simulink model "LinearCompetitiveModel"  (R2023b)
settings: Solver=FixedStepAuto  StartTime=0.0  StopTime=inf  RelTol=1e-3
undefined symbols (not defined in the file or in its folder): DiscIntNeverNeededParam
libraries: arduinolib x14, simulink x12, mobileRoboticsTrainingLib x1, arduinosensorlib x1
settings Model: ExtModeTrigDuration=2  Creator=cameronclark  LastModifiedBy=cameronclark
settings OptimizationCC: EnhancedBackFolding=on  PassReuseOutputArgsAs=Individual arguments  ZeroExternalMemoryAtStartup=off  ZeroInternalMemoryAtStartup=off  MaxStackSize=64  OptimizeBlockOrder=speed  DifferentSizesBufferReuse=on  OptimizationCustomize=off  EfficientTunableParamExpr=on
settings DebuggingCC: ParameterTunabilityLossMsg=error
settings HardwareCC: ProdBitPerPointer=32  ProdBitPerSizeT=32  ProdBitPerPtrDiffT=32  ProdLargestAtomicInteger=Long  ProdLargestAtomicFloat=Double  ProdWordSize=32  ProdHWDeviceType=ARM Compatible->ARM Cortex  UseEmbeddedCoderFeatures=off  UseSimulinkCoderFeatures=off
settings SFSimCC: MATLABDynamicMemAlloc=off
settings RTWCC: Description=Embedded Coder  SystemTargetFile=ert.tlc  HardwareBoard=Arduino Nano 33 IoT  TemplateMakefile=ert_default_tmf  Toolchain=Arduino ARM  BuildConfiguration=Faster Runs
settings CodeAppCC: ForceParamTrailComments=on  IgnoreCustomStorageClasses=off  OperatorAnnotations=on  SimulinkDataObjDesc=on  SFDataObjDesc=on  InsertBlockDesc=on
settings ERTTargetCC: SupportContinuousTime=on  SupportNonInlinedSFcns=on  SupportVariableSizeSignals=on  ExtModeTransport=3  ExtModeStaticAlloc=on  ExtModeAutomaticAllocSize=off  ExtModeStaticAllocSize=8192  ExtModeMexFile=ext_xcp  ExtModeIntrfLevel=Level2 - Open

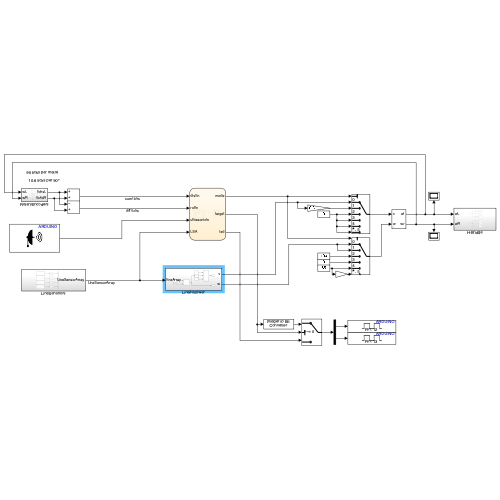
[thumbnail: Simulink's stored preview of the top-level diagram]
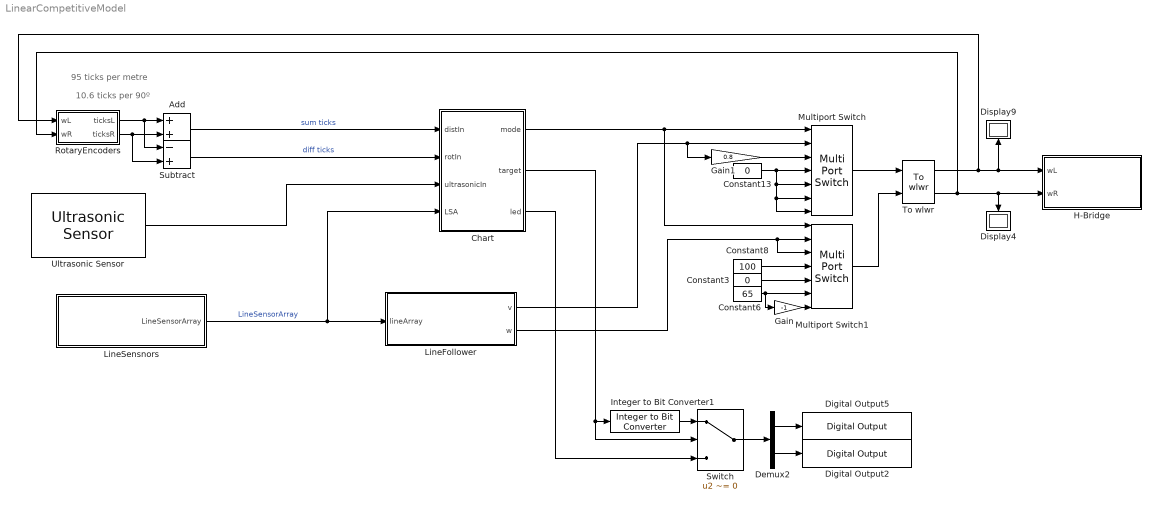
== system LinearCompetitiveModel ==
  note: 95 ticks per metre
  note: 10.6 ticks per 90º
  Add : Sum
  Chart : Stateflow chart  TreatAsAtomicUnit=on
  Constant13 : Constant  Value=0
  Constant3 : Constant  Value=0
  Constant6 : Constant  Value=65
  Constant8 : Constant  Value=100
  Demux2 : Demux  Outputs=2
  Digital Output2 : arduinolib/Digital Output  pinNumber=13  Direction=output  blockPlatform=arduino
  Digital Output5 : arduinolib/Digital Output  pinNumber=12  Direction=output  blockPlatform=arduino
  Display4 : Display
  Display9 : Display
  Gain : Gain  Gain=-1
  Gain1 : Gain  Gain=0.8
  H-Bridge : Subsystem
  Integer to Bit Converter1 : simulink/Logic and Bit Operations/Integer to Bit Converter  nbits=2  signedInputValues=Unsigned  bitOrder=MSB first  outDtype=Inherit via internal rule
  LineFollower : Subsystem
  LineSensnors : Subsystem
  Multiport Switch : MultiPortSwitch  DataPortOrder=Zero-based contiguous  Inputs=6  DataPortIndices={0,1,3,4}  zeroidx=on  SaturateOnIntegerOverflow=off
  Multiport Switch1 : MultiPortSwitch  DataPortOrder=Zero-based contiguous  Inputs=6  DataPortIndices={0,1,3,4}  zeroidx=on  SaturateOnIntegerOverflow=off  InputSameDT=off
  RotaryEncoders : Subsystem
  Subtract : Sum  Inputs=-+
  Switch : Switch  Criteria=u2 ~= 0  SaturateOnIntegerOverflow=off  InputSameDT=off
  To wlwr : mobileRoboticsTrainingLib/To wlwr  axleLength=0.1  wheelR=0.05
      link override change parameters: Gain=[1 -axleLength/2;1 axleLength/2]
  Ultrasonic Sensor : arduinosensorlib/Ultrasonic Sensor  NumSignalPins=2  TrigPin=8  EchoPin=11  SignalPin=3  SampleTime_=0.1  blockPlatform=ARDUINO
  wires:
  RotaryEncoders/2(ticksR) -> Subtract/2, Add/2
  Subtract/1 -> Chart/2(rotIn)  "diff ticks"
  Multiport Switch/1 -> To wlwr/1
  To wlwr/2 -> RotaryEncoders/2(wR), H-Bridge/2(wR), Display4/1
  LineSensnors/1(LineSensorArray) -> LineFollower/1(lineArray), Chart/4(LSA)  "LineSensorArray"
  Constant8/1 -> Multiport Switch1/4
  Multiport Switch1/1 -> To wlwr/2
  Constant6/1 -> Gain/1, Multiport Switch1/6
  LineFollower/1(v) -> Multiport Switch/2, Gain1/1
  Gain/1 -> Multiport Switch1/7
  RotaryEncoders/1(ticksL) -> Subtract/1, Add/1
  Chart/1(mode) -> Multiport Switch/1, Multiport Switch1/1
  Constant3/1 -> Multiport Switch1/5
  LineFollower/2(w) -> Multiport Switch1/2, Multiport Switch1/3
  Ultrasonic Sensor/1 -> Chart/3(ultrasonicIn)
  Constant13/1 -> Multiport Switch/7, Multiport Switch/6, Multiport Switch/5, Multiport Switch/4
  To wlwr/1 -> RotaryEncoders/1(wL), H-Bridge/1(wL), Display9/1
  Add/1 -> Chart/1(distIn)  "sum ticks"
  Demux2/2 -> Digital Output2/1
  Demux2/1 -> Digital Output5/1
  Switch/1 -> Demux2/1
  Gain1/1 -> Multiport Switch/3
  Chart/2(target) -> Integer to Bit Converter1/1, Switch/2
  Chart/3(led) -> Switch/3
  Integer to Bit Converter1/1 -> Switch/1

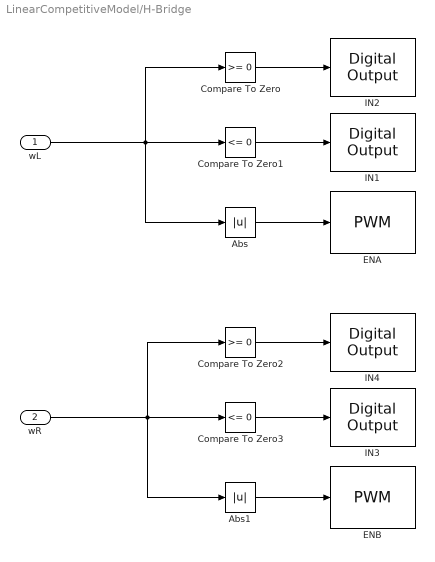
== system LinearCompetitiveModel/H-Bridge ==
  wL : Inport
  wR : Inport  Port=2
  Abs : Abs  SaturateOnIntegerOverflow=off
  Abs1 : Abs  SaturateOnIntegerOverflow=off
  Compare To Zero : simulink/Logic and Bit Operations/Compare To Zero  relop=>=  OutDataTypeStr=boolean
  Compare To Zero1 : simulink/Logic and Bit Operations/Compare To Zero  relop=<=  OutDataTypeStr=boolean
  Compare To Zero2 : simulink/Logic and Bit Operations/Compare To Zero  relop=>=  OutDataTypeStr=boolean
  Compare To Zero3 : simulink/Logic and Bit Operations/Compare To Zero  relop=<=  OutDataTypeStr=boolean
  ENA : arduinolib/PWM  pinNumber=4  frequencyType=Default  desiredFrequency=490.2  achievableFrequency=490.2
  ENB : arduinolib/PWM  pinNumber=5  frequencyType=Default  desiredFrequency=490.2  achievableFrequency=490.2
  IN1 : arduinolib/Digital Output  pinNumber=2  Direction=output  blockPlatform=arduino
  IN2 : arduinolib/Digital Output  pinNumber=3  Direction=output  blockPlatform=arduino
  IN3 : arduinolib/Digital Output  pinNumber=6  Direction=output  blockPlatform=arduino
  IN4 : arduinolib/Digital Output  pinNumber=7  Direction=output  blockPlatform=arduino
  wires:
  Compare To Zero1/1 -> IN1/1
  Compare To Zero/1 -> IN2/1
  Abs1/1 -> ENB/1
  Compare To Zero3/1 -> IN3/1
  Compare To Zero2/1 -> IN4/1
  wL/1 -> Compare To Zero/1, Compare To Zero1/1, Abs/1
  Abs/1 -> ENA/1
  wR/1 -> Compare To Zero2/1, Compare To Zero3/1, Abs1/1

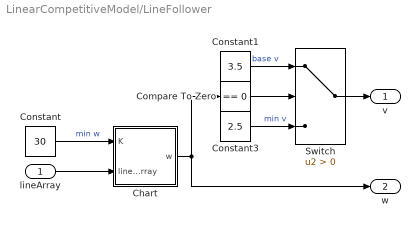
== system LinearCompetitiveModel/LineFollower ==
  lineArray : Inport
  Chart : Stateflow chart  TreatAsAtomicUnit=on
  Compare To Zero : simulink/Logic and Bit Operations/Compare To Zero  relop===  OutDataTypeStr=boolean
  Constant : Constant  Value=30
  Constant1 : Constant  Value=3.5
  Constant3 : Constant  Value=2.5
  Switch : Switch  Criteria=u2 > Threshold  SaturateOnIntegerOverflow=off  InputSameDT=off
  v : Outport
  w : Outport  Port=2
  wires:
  Constant1/1 -> Switch/1  "base v"
  Chart/1(w) -> Compare To Zero/1, w/1
  Constant3/1 -> Switch/3  "min v"
  Switch/1 -> v/1
  lineArray/1 -> Chart/2(lineArray)
  Compare To Zero/1 -> Switch/2
  Constant/1 -> Chart/1(K)  "min w"

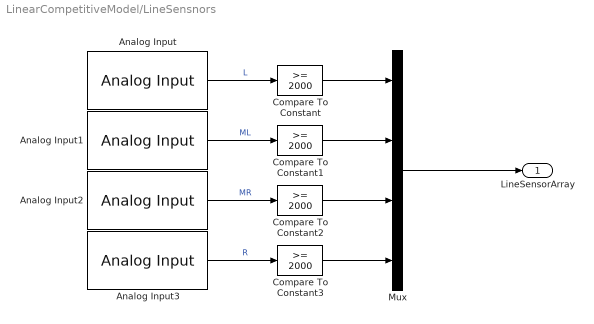
== system LinearCompetitiveModel/LineSensnors ==
  Analog Input : arduinolib/Analog Input  pinNumber=7  ReadResultsOnly=off  ConversionTriggerSource=Software  ExternalTriggerType=uint32( 0 )  OutputDataType=uint16  EnableConversionCompleteNotify=off  EnableOuputStatus=off  SampleTime=-1  blockPlatform=arduino
  Analog Input1 : arduinolib/Analog Input  pinNumber=6  ReadResultsOnly=off  ConversionTriggerSource=Software  ExternalTriggerType=uint32( 0 )  OutputDataType=uint16  EnableConversionCompleteNotify=off  EnableOuputStatus=off  SampleTime=-1  blockPlatform=arduino
  Analog Input2 : arduinolib/Analog Input  pinNumber=3  ReadResultsOnly=off  ConversionTriggerSource=Software  ExternalTriggerType=uint32( 0 )  OutputDataType=uint16  EnableConversionCompleteNotify=off  EnableOuputStatus=off  SampleTime=-1  blockPlatform=arduino
  Analog Input3 : arduinolib/Analog Input  pinNumber=2  ReadResultsOnly=off  ConversionTriggerSource=Software  ExternalTriggerType=uint32( 0 )  OutputDataType=uint16  EnableConversionCompleteNotify=off  EnableOuputStatus=off  SampleTime=-1  blockPlatform=arduino
  Compare To Constant{,1..3} (4 alike) : simulink/Logic and Bit Operations/Compare To Constant  relop=>=  const=2000  OutDataTypeStr=boolean
  Mux : Mux
  LineSensorArray : Outport
  wires:
  Mux/1 -> LineSensorArray/1
  Analog Input/1 -> Compare To Constant/1  "L"
  Analog Input1/1 -> Compare To Constant1/1  "ML"
  Analog Input2/1 -> Compare To Constant2/1  "MR"
  Analog Input3/1 -> Compare To Constant3/1  "R"
  Compare To Constant/1 -> Mux/1
  Compare To Constant1/1 -> Mux/2
  Compare To Constant2/1 -> Mux/3
  Compare To Constant3/1 -> Mux/4

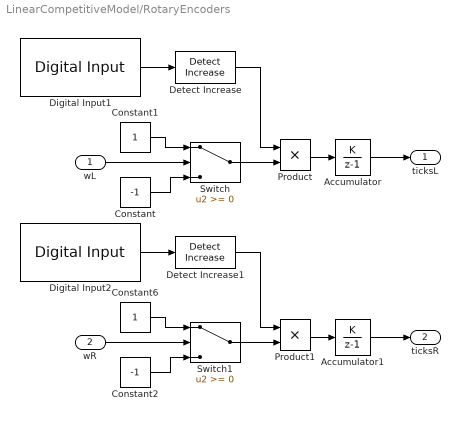
== system LinearCompetitiveModel/RotaryEncoders ==
  wL : Inport
  wR : Inport  Port=2
  Accumulator : DiscreteIntegrator  IntegratorMethod=Accumulation: Forward Euler  SampleTime=-1  ICPrevOutput=DiscIntNeverNeededParam  ICPrevScaledInput=DiscIntNeverNeededParam
  Accumulator1 : DiscreteIntegrator  IntegratorMethod=Accumulation: Forward Euler  SampleTime=-1  ICPrevOutput=DiscIntNeverNeededParam  ICPrevScaledInput=DiscIntNeverNeededParam
  Constant : Constant  Value=-1
  Constant1 : Constant
  Constant2 : Constant  Value=-1
  Constant6 : Constant
  Detect Increase : simulink/Logic and Bit Operations/Detect Increase  vinit=0.0  OutDataTypeStr=boolean
  Detect Increase1 : simulink/Logic and Bit Operations/Detect Increase  vinit=0.0  OutDataTypeStr=boolean
  Digital Input1 : arduinolib/Digital Input  pinNumber=9  mode=Default  Direction=input  SampleTime=0.1  blockPlatform=arduino
  Digital Input2 : arduinolib/Digital Input  pinNumber=10  mode=Default  Direction=input  SampleTime=0.1  blockPlatform=arduino
  Product : Product
  Product1 : Product
  Switch : Switch  SaturateOnIntegerOverflow=off  InputSameDT=off
  Switch1 : Switch  SaturateOnIntegerOverflow=off  InputSameDT=off
  ticksL : Outport
  ticksR : Outport  Port=2
  wires:
  wL/1 -> Switch/2
  Constant1/1 -> Switch/1
  Constant/1 -> Switch/3
  Digital Input1/1 -> Detect Increase/1
  Switch/1 -> Product/2
  Accumulator/1 -> ticksL/1
  wR/1 -> Switch1/2
  Constant6/1 -> Switch1/1
  Constant2/1 -> Switch1/3
  Accumulator1/1 -> ticksR/1
  Switch1/1 -> Product1/2
  Product/1 -> Accumulator/1
  Detect Increase/1 -> Product/1
  Detect Increase1/1 -> Product1/1
  Digital Input2/1 -> Detect Increase1/1
  Product1/1 -> Accumulator1/1

== stateflow chart LinearCompetitiveModel/LineFollower/Chart ==
  state ComputeW
    %code for the line array
    during:
    w = K*(lineArray(3)-lineArray(2));
  (default) -> ComputeW
  data: w output; K input; lineArray input

== stateflow chart LinearCompetitiveModel/Chart ==
  state Setup
    entry:
    intersections = zeros(10);
    intersection = 0;
  state Explore
    state Explore
      entry:
      mode = 0;
      led = [0 0];
    state TurnBackOffLine
      entry:
      mode = 4 + turn;
    state TurnBackOntoLine
    state CentreBackOffIntersection
      entry:
      mode = 1;
      distT = distIn + 5;
    state CentreOnIntersection
      entry:
      mode = 1;
      distT = distIn + 5;
    state SharpTurn
      entry:
      mode = 4 + turn;
    state DriveBackToInterection
      entry:
      mode = 0;
    state TurnOffLine
      entry:
      mode = 4 + turn;
    state TurnAround
      entry:
      mode = 4;
      rotT = rotIn + 14;
    state TurnOntoLine
    state DeadEnd
      entry:
      intersection = intersection + 1;
      intersections(intersection) = 2;
    state MoveForward
      entry:
      mode = 1;
      distT = distIn + 5
    state DriveToEnd
      entry:
      mode=0;
    state UltrasonicSense
      entry:
      mode=3;
      exit:
      intersection = intersection + 1;
      intersections(intersection) = ultrasonicIn;
      led = [1 (ultrasonicIn < 0.15)];
    TurnBackOntoLine -> Explore.Explore : [LSA(2)==0 & LSA(3)==0]
    Explore.SharpTurn -> Explore.Explore : [LSA(2)==0 & LSA(3)==0]
    Explore.Explore -> Explore.CentreOnIntersection [order 1] : [LSA(1)==0]
        | {turn=0;}
    Explore.Explore -> Explore.CentreOnIntersection [order 2] : [LSA(4)==0]
        | {turn=1;}
    TurnBackOffLine -> TurnBackOntoLine : [LSA(2)==1 & LSA(3)==1]
    CentreBackOffIntersection -> TurnBackOffLine : [distIn>=distT]
    Explore.CentreOnIntersection -> Explore.SharpTurn [order 3] : [LSA(2)==1 & LSA(3)==1]
    DriveBackToInterection -> CentreBackOffIntersection : [LSA(1)==0 | LSA(4) == 0]
    Explore.CentreOnIntersection -> Explore.TurnOffLine [order 2] : [distIn>=distT]
    Explore.TurnAround -> DriveBackToInterection : [rotIn>rotT & LSA(3)==0]
    Explore.TurnOffLine -> Explore.TurnOntoLine : [LSA(2)==1 & LSA(3)==1]
    Explore.TurnOntoLine -> Explore.DriveToEnd : [LSA(2)==0 & LSA(3)==0]
    MoveForward -> Explore.TurnAround : [distIn>=distT]
    Explore.DriveToEnd -> DeadEnd [order 2] : [all(LSA==1)]
    DeadEnd -> MoveForward
    Explore.DriveToEnd -> UltrasonicSense [order 1] : [LSA(1)==0 & LSA(4)==0]
    UltrasonicSense -> MoveForward : after(300, msec)
  state Return
    state Return
      entry:
      mode = 0;
    state CentreOnIntersection
      entry:
      mode = 1;
      distT = distIn + 5;
    state SharpTurn
      entry:
      mode = 4 + turn;
    state Stop
      entry:
      mode = 3;
    state Count
      exit:
      target = target - 1;
    state TurnOffLine
      entry:
      mode = 4 + turn;
    state SPIIIIINNN
      entry:
      mode = 2;
    state DriveToEnd
      entry:
      mode=1;
    state Wait
      entry:
      mode = 3;
    state TurnOntoLine
    Return.SharpTurn -> Return.Return : [LSA(2)==0 & LSA(3)==0]
    Return.Return -> Return.CentreOnIntersection [order 1] : [LSA(1)==0]
        | {turn=0;}
    Return.Return -> Return.CentreOnIntersection [order 2] : [LSA(4)==0]
        | {turn=1;}
    Count -> Return.Return [order 2] : [LSA(1)==1 & LSA(4)==1]
    Return.CentreOnIntersection -> Return.SharpTurn [order 1] : [LSA(2)==1 & LSA(3)==1]
    Return.CentreOnIntersection -> Count [order 2] : [distIn>=distT]
    Count -> Return.TurnOffLine [order 1] : [target==0]
    SPIIIIINNN -> Stop : after(5,sec)
    Return.TurnOffLine -> Return.TurnOntoLine : [LSA(2)==1 & LSA(3)==1]
    Wait -> SPIIIIINNN : after(2,sec)
    Return.TurnOntoLine -> Return.DriveToEnd : [LSA(2)==0 & LSA(3)==0]
    Return.DriveToEnd -> Wait : [LSA(1)==0 | LSA(4)==0]
  state TurnAround
    entry:
    mode = 4;
    rotT = rotIn + 14;
  state TargetObject
    entry:
    closestObj = 2;
    for target = 1:intersection
    if intersections(target) < closestObj
    closestObj = intersections(target);
    end
    end
    for target = 1:intersection
    if intersections(target) == closestObj
    break;
    end
    end
    target = intersection - target;
  (default) -> Setup
  Setup -> Explore.Explore
  TurnAround -> Return.Return : [rotIn>rotT & LSA(3)==0]
  TargetObject -> TurnAround
  Explore.CentreOnIntersection -> TargetObject [order 1] : [LSA(1)==0 & LSA(4)==0]
  data: distIn input; rotIn input; mode output; ultrasonicIn input; LSA input; distT local; rotT local; intersections local; intersection local; turn local; closestObj local; target output; led output
